simulink subsystem "WSS"  (R2025b)
settings: Solver=VariableStepAuto  StartTime=0.0  StopTime=10.0  RelTol=1e-3
libraries: simulink x1
settings Model: Creator=diego  LastModifiedBy=diego

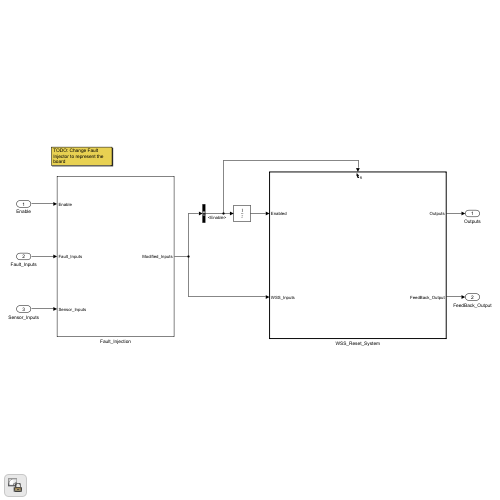
[thumbnail: Simulink's stored preview of the top-level diagram]
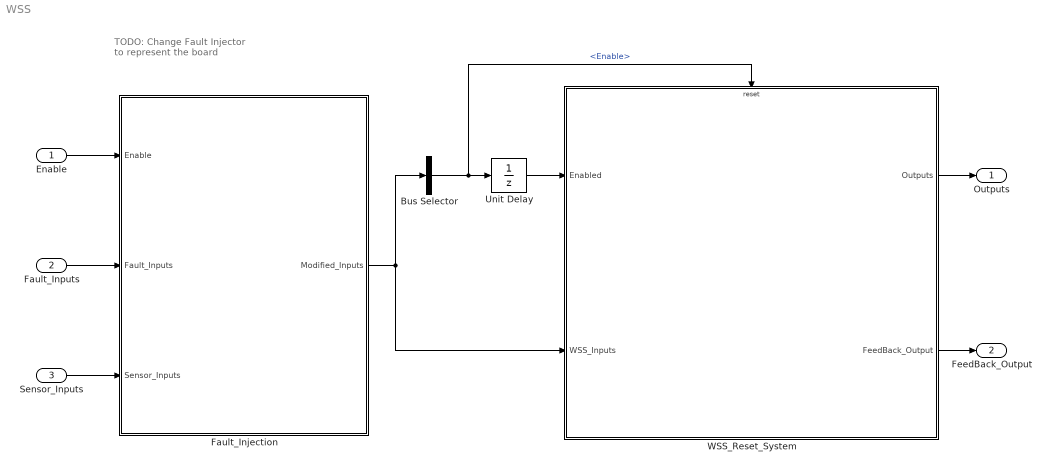
== system WSS ==
  note: TODO: Change Fault Injector to represent the board
  Enable : Inport
  Fault_Inputs : Inport  Port=2
  Sensor_Inputs : Inport  Port=3
  Bus Selector : BusSelector  OutputSignals=Enable
  Fault_Injection : Subsystem
  Unit Delay : UnitDelay  SampleTime=-1  HasFrameUpgradeWarning=on
  "WSS_Reset_System " : Subsystem  TreatAsAtomicUnit=on
  Outputs : Outport
  FeedBack_Output : Outport  Port=2
  wires:
  "WSS_Reset_System "/1(Outputs) -> Outputs/1
  Fault_Injection/1(Modified_Inputs) -> "WSS_Reset_System "/2(WSS_Inputs), Bus Selector/1
  Bus Selector/1 -> Unit Delay/1, "WSS_Reset_System "/Reset  "<Enable>"
  Fault_Inputs/1 -> Fault_Injection/2(Fault_Inputs)
  Enable/1 -> Fault_Injection/1(Enable)
  Unit Delay/1 -> "WSS_Reset_System "/1(Enabled)
  Sensor_Inputs/1 -> Fault_Injection/3(Sensor_Inputs)
  "WSS_Reset_System "/2(FeedBack_Output) -> FeedBack_Output/1

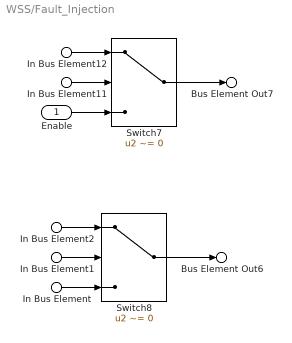
== system WSS/Fault_Injection ==
  Enable : Inport
  In Bus Element12 : Inport  Port=2  PortName=Fault_Inputs  Element=Acc_EN
  In Bus Element11 : Inport  Port=2  PortName=Fault_Inputs  Element=Override_Acc_EN
  In Bus Element1 : Inport  Port=2  PortName=Fault_Inputs  Element=Override_Wheel_Speed
  In Bus Element2 : Inport  Port=2  PortName=Fault_Inputs  Element=Wheel_Speed
  In Bus Element : Inport  Port=3  PortName=Sensor_Inputs  Element=WSS_Wheel_Speed
  Switch7 : Switch  Criteria=u2 ~= 0  SaturateOnIntegerOverflow=off  InputSameDT=off
  Switch8 : Switch  Criteria=u2 ~= 0  SaturateOnIntegerOverflow=off  InputSameDT=off
  Bus Element Out7 : Outport  PortName=Modified_Inputs  Element=Enable
  Bus Element Out6 : Outport  PortName=Modified_Inputs  Element=Wheel_Speed
  wires:
  In Bus Element2/1 -> Switch8/1
  Switch8/1 -> Bus Element Out6/1
  In Bus Element/1 -> Switch8/3
  In Bus Element1/1 -> Switch8/2
  In Bus Element12/1 -> Switch7/1
  Switch7/1 -> Bus Element Out7/1
  In Bus Element11/1 -> Switch7/2
  Enable/1 -> Switch7/3

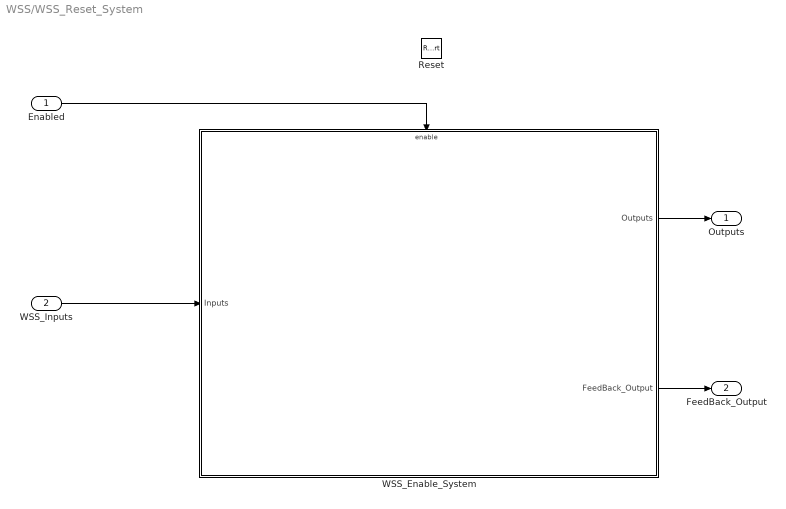
== system WSS/WSS_Reset_System  ==
  Enabled : Inport
  WSS_Inputs : Inport  Port=2
  Reset : ResetPort  DisableCoverage=on  ResetTriggerType=falling
  "WSS_Enable_System " : Subsystem  TreatAsAtomicUnit=on
  Outputs : Outport
  FeedBack_Output : Outport  Port=2
  wires:
  "WSS_Enable_System "/2(FeedBack_Output) -> FeedBack_Output/1
  "WSS_Enable_System "/1(Outputs) -> Outputs/1
  WSS_Inputs/1 -> "WSS_Enable_System "/1(Inputs)
  Enabled/1 -> "WSS_Enable_System "/Enable

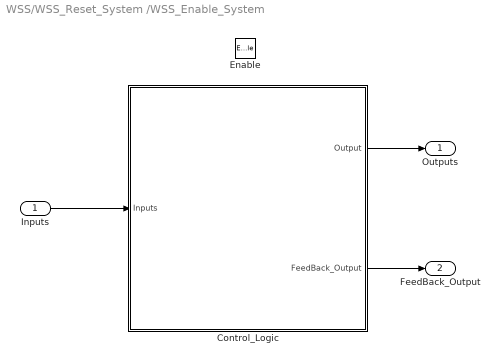
== system WSS/WSS_Reset_System /WSS_Enable_System  ==
  Inputs : Inport
  Enable : EnablePort  StatesWhenEnabling=reset
  Control_Logic : Subsystem
  Outputs : Outport
  FeedBack_Output : Outport  Port=2
  wires:
  Control_Logic/2(FeedBack_Output) -> FeedBack_Output/1
  Control_Logic/1(Output) -> Outputs/1
  Inputs/1 -> Control_Logic/1(Inputs)

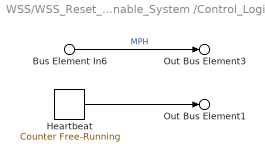
== system WSS/WSS_Reset_System /WSS_Enable_System /Control_Logic ==
  Bus Element In6 : Inport  PortName=Inputs  Element=Wheel_Speed
  Heartbeat : simulink/Sources/Counter Free-Running  NumBits=32  tsamp=-1
  Out Bus Element3 : Outport  PortName=Output  Element=WSS_Wheel_Speed
  Out Bus Element1 : Outport  Port=2  PortName=FeedBack_Output  Element=WSS_Heartbeat
  wires:
  Bus Element In6/1 -> Out Bus Element3/1  "MPH"
  Heartbeat/1 -> Out Bus Element1/1
